simulink model "Q1_b"  (R2020b)
settings: Solver=VariableStepAuto  StartTime=0.0  StopTime=60.0  RelTol=1e-3
settings Model: Creator=aloks  LastModifiedBy=aloks

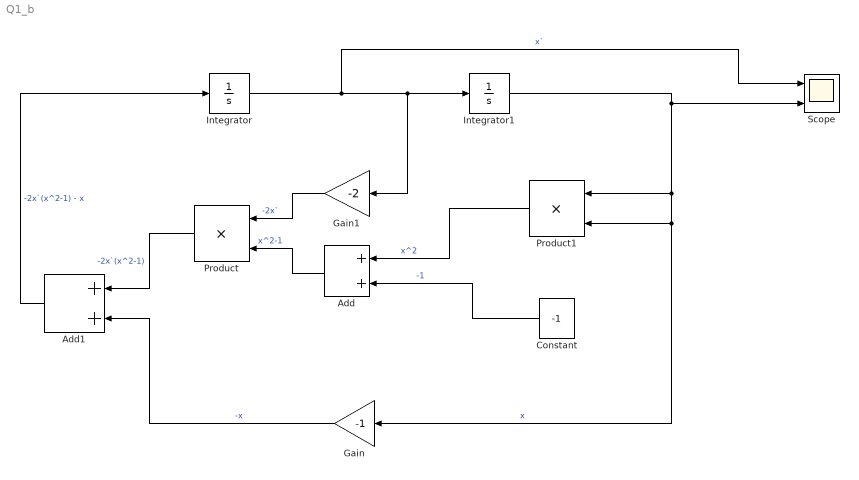
== system Q1_b ==
  Add : Sum
  Add1 : Sum
  Constant : Constant  Value=-1
  Gain : Gain  Gain=-1
  Gain1 : Gain  Gain=-2
  Integrator : Integrator  InitialCondition=0.1
  Integrator1 : Integrator
  Product : Product
  Product1 : Product
  Scope : Scope  NumInputPorts=2
  wires:
  Integrator/1 -> Scope/1, Gain1/1, Integrator1/1  "x`"
  Integrator1/1 -> Product1/1, Product1/2, Gain/1, Scope/2  "x"
  Constant/1 -> Add/2  "-1"
  Add/1 -> Product/2  "x^2-1"
  Gain1/1 -> Product/1  "-2x`"
  Gain/1 -> Add1/2  "-x"
  Product/1 -> Add1/1  "-2x`(x^2-1)"
  Add1/1 -> Integrator/1  "-2x`(x^2-1) - x"
  Product1/1 -> Add/1  "x^2"
